simulink model "problem1"  (R2020b)
settings: Solver=VariableStepAuto  StartTime=0.0  StopTime=10.0  RelTol=1e-3
settings Model: Creator=Hp  LastModifiedBy=Hp

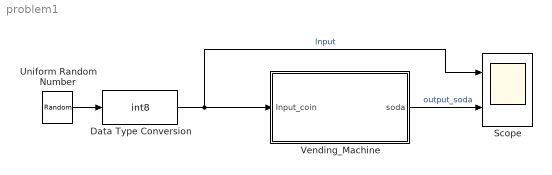
== system problem1 ==
  Data Type Conversion : DataTypeConversion  OutDataTypeStr=int8  RndMeth=Nearest  SaturateOnIntegerOverflow=on
  Scope : Scope  NumInputPorts=2
  Uniform Random Number : UniformRandomNumber  Minimum=0  Maximum=4  Seed=337  SampleTime=0.1
  Vending_Machine : Stateflow chart  TreatAsAtomicUnit=on
  wires:
  Vending_Machine/1(soda) -> Scope/2  "output_soda"
  Data Type Conversion/1 -> Vending_Machine/1(Input_coin), Scope/1  "Input"
  Uniform Random Number/1 -> Data Type Conversion/1

== stateflow chart problem1/Vending_Machine ==
  settings: stateMachineType=MEALY_MACHINE  initializeOutput=1
  state Initial_state
  state State_nickel
  state State_dime
  (default) -> Initial_state
  Initial_state -> State_nickel [order 1] : [Input_coin==1]{soda=0}
  State_nickel -> Initial_state [order 2] : [Input_coin==2]{soda=1}
  State_dime -> Initial_state [order 1] : [Input_coin==1]{soda=1}
  Initial_state -> State_dime [order 2] : [Input_coin==2]{soda=0}
  State_nickel -> State_dime [order 1] : [Input_coin==1]{soda=0}
  State_dime -> State_nickel [order 2] : [Input_coin==2]{soda=1}
  data: Input_coin input int8; soda output boolean
